simulink model "ejemplo1"  (R2019a)
settings: Solver=VariableStepAuto  StartTime=0.0  StopTime=50  RelTol=1e-3
values from neighbouring files (symbols this model uses):
  b = 4    [simulacion.m]
  k = 2    [simulacion.m]
  m = 10    [simulacion.m]
settings Model: Creator=cmparedes  LastModifiedBy=cmparedes

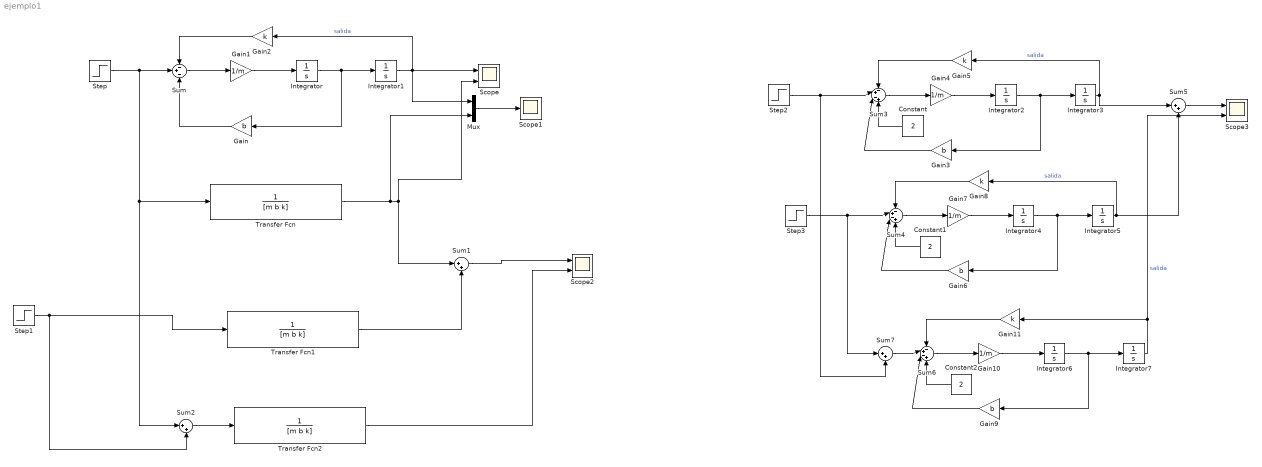
== system ejemplo1 ==
  Constant : Constant  Value=2
  Constant1 : Constant  Value=2
  Constant2 : Constant  Value=2
  Gain{,3,6,9} (4 alike) : Gain  Gain=b
  Gain{1,4,7,10} (4 alike) : Gain  Gain=1/m
  Gain{2,5,8,11} (4 alike) : Gain  Gain=k
  Integrator{,1..7} (8 alike) : Integrator
  Mux : Mux  Inputs=2
  Scope : Scope  NumInputPorts=2
  Scope1 : Scope
  Scope2 : Scope  NumInputPorts=2
  Scope3 : Scope  NumInputPorts=2
  Step : Step  Time=0  After=-3  SampleTime=0
  Step1 : Step  Time=0  After=2  SampleTime=0
  Step2 : Step  Time=0  After=-3  SampleTime=0
  Step3 : Step  Time=0  After=4  SampleTime=0
  Sum : Sum  Inputs=-+-
  Sum{1..2,5,7} (4 alike) : Sum  Inputs=|++
  Sum3 : Sum  Inputs=-+-+
  Sum4 : Sum  Inputs=-+-+
  Sum6 : Sum  Inputs=-+-+
  Transfer Fcn : TransferFcn  Numerator=1  Denominator=[m b k]
  Transfer Fcn1 : TransferFcn  Numerator=1  Denominator=[m b k]
  Transfer Fcn2 : TransferFcn  Numerator=1  Denominator=[m b k]
  wires:
  Sum/1 -> Gain1/1
  Gain1/1 -> Integrator/1
  Integrator/1 -> Gain/1, Integrator1/1
  Gain/1 -> Sum/3
  Gain2/1 -> Sum/1
  Step/1 -> Sum2/1, Transfer Fcn/1, Sum/2
  Integrator1/1 -> Gain2/1, Scope/1, Mux/1  "salida"
  Transfer Fcn/1 -> Mux/2, Sum1/1, Scope/2
  Mux/1 -> Scope1/1
  Step1/1 -> Sum2/2, Transfer Fcn1/1
  Transfer Fcn1/1 -> Sum1/2
  Sum1/1 -> Scope2/1
  Sum2/1 -> Transfer Fcn2/1
  Transfer Fcn2/1 -> Scope2/2
  Gain5/1 -> Sum3/1
  Gain3/1 -> Sum3/3
  Integrator2/1 -> Gain3/1, Integrator3/1
  Sum3/1 -> Gain4/1
  Gain4/1 -> Integrator2/1
  Step2/1 -> Sum7/2, Sum3/2
  Integrator3/1 -> Gain5/1, Sum5/1  "salida"
  Constant/1 -> Sum3/4
  Step3/1 -> Sum7/1, Sum4/2
  Constant1/1 -> Sum4/4
  Integrator5/1 -> Sum5/2, Gain8/1  "salida"
  Sum4/1 -> Gain7/1
  Gain6/1 -> Sum4/3
  Gain7/1 -> Integrator4/1
  Gain8/1 -> Sum4/1
  Integrator4/1 -> Gain6/1, Integrator5/1
  Sum5/1 -> Scope3/1
  Sum7/1 -> Sum6/2
  Constant2/1 -> Sum6/4
  Integrator7/1 -> Scope3/2, Gain11/1  "salida"
  Sum6/1 -> Gain10/1
  Gain9/1 -> Sum6/3
  Gain10/1 -> Integrator6/1
  Gain11/1 -> Sum6/1
  Integrator6/1 -> Gain9/1, Integrator7/1
